simulink model "aydinuzun1"  (R2016b)
settings: Solver=VariableStepAuto  StartTime=0.0  StopTime=10.0  RelTol=1e-3
settings Model: Creator=aydn  LastModifiedBy=aydn

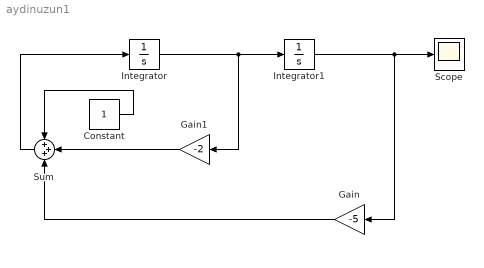
== system aydinuzun1 ==
  Constant : Constant
  Gain : Gain  Gain=-5
  Gain1 : Gain  Gain=-2
  Integrator : Integrator  InitialCondition=0.05
  Integrator1 : Integrator  InitialCondition=0.1
  Scope : Scope
  Sum : Sum  Inputs=3
  wires:
  Integrator/1 -> Gain1/1, Integrator1/1
  Integrator1/1 -> Gain/1, Scope/1
  Gain1/1 -> Sum/2
  Gain/1 -> Sum/3
  Constant/1 -> Sum/1
  Sum/1 -> Integrator/1
